simulink model "bh_COMPONENT_3dof_4wheel_car_model"  (R2018a)
settings: Solver=ode45  StartTime=0.0  StopTime=80  FixedStep=0.001  RelTol=1e-5
undefined symbols (not defined in the file): veh, VwW_X_b_L, VwW_X_b_R, VwW_X_f_L, VwW_X_f_R
settings Model: PauseTimes=30  Creator=bhorton  LastModifiedBy=bhorton
settings SolverCC: ZeroCrossControl=EnableAll  ZeroCrossAlgorithm=Adaptive
settings DebuggingCC: SignalInfNanChecking=warning

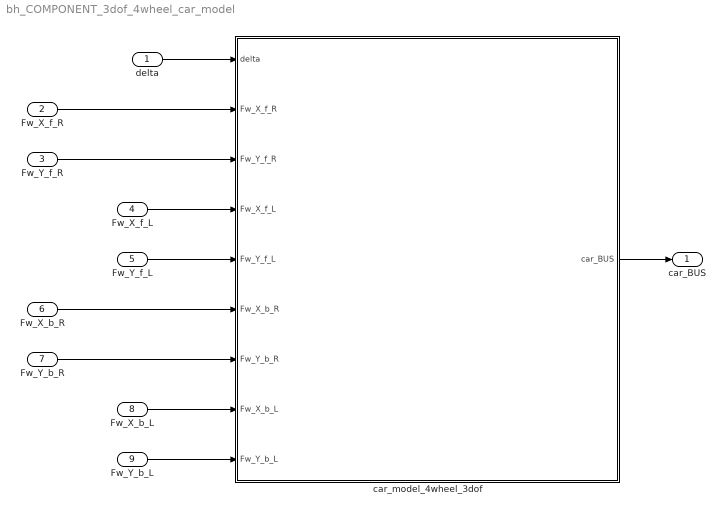
== system bh_COMPONENT_3dof_4wheel_car_model ==
  delta : Inport
  Fw_X_f_R : Inport  Port=2
  Fw_Y_f_R : Inport  Port=3
  Fw_X_f_L : Inport  Port=4
  Fw_Y_f_L : Inport  Port=5
  Fw_X_b_R : Inport  Port=6
  Fw_Y_b_R : Inport  Port=7
  Fw_X_b_L : Inport  Port=8
  Fw_Y_b_L : Inport  Port=9
  car_model_4wheel_3dof : Subsystem  mask{L_f=veh.Lf, L_b=veh.Lb, L_p=veh.Lp, L_d=veh.Ld, m=veh.mass, I_zz=veh.Inertia, v_xB_0=veh.states.init_vel_B_Cx, v_yB_0=veh.states.init_vel_B_Cy, xG_0=veh.states.init_pos_G_Cxy(1), yG_0=veh.states.init_pos_G_Cxy(2), theta_D_0=veh.states.init_theta_vel_rad, theta_0=veh.states.init_theta_pos_rad}
      mask prompts: L_f "Lf  (m)"; L_b "Lb  (m)"; L_p "Lp  (m)"; L_d "Ld  (m)"; m "m  (kg)"; I_zz "I_zz (kg.m^2)"; v_xB_0 "vB_X  (m/sec)"; v_yB_0 "vB_Y (m/sec)"; xG_0 "xG_0 (m)"; yG_0 "yG_0 (m)"; theta_D_0 "theta_dot_0 (rad/sec)"; theta_0 "theta_0  (rad)"
      mask DialogControl DescGroupVar Prompt: 3-dof_4wheel_car_dynamics
      mask DialogControl DescTextVar Prompt: 3-dof 4 wheel car model
      mask DialogControl Container7 Prompt: Diagrams
      mask DialogControl Container12 Prompt: 01
      mask DialogControl Container14 Prompt: 02
      mask DialogControl Container15 Prompt: 03
      mask DialogControl Container24 Prompt: 04
      mask DialogControl Container25 Prompt: 05
      mask DialogControl Container9 Prompt: Geometry
      mask DialogControl Container10 Prompt: Mass
      mask DialogControl Container13 Prompt: States
      mask DialogControl Control5 Prompt: INITIAL velocity in BODY {B}-frame
      mask DialogControl Control6 Prompt: INITIAL position in INERTIAL {G}-frame
      mask DialogControl Control4 Prompt: INITIAL Angular states:
      mask Display: image(imread('bh_CAR_geo_07.JPG'), 'center')
  car_BUS : Outport  OutDataTypeStr=Bus: car_BUS
  wires:
  car_model_4wheel_3dof/1(car_BUS) -> car_BUS/1
  Fw_X_b_L/1 -> car_model_4wheel_3dof/8(Fw_X_b_L)
  Fw_Y_b_L/1 -> car_model_4wheel_3dof/9(Fw_Y_b_L)
  Fw_X_f_R/1 -> car_model_4wheel_3dof/2(Fw_X_f_R)
  Fw_Y_b_R/1 -> car_model_4wheel_3dof/7(Fw_Y_b_R)
  Fw_X_b_R/1 -> car_model_4wheel_3dof/6(Fw_X_b_R)
  Fw_X_f_L/1 -> car_model_4wheel_3dof/4(Fw_X_f_L)
  Fw_Y_f_L/1 -> car_model_4wheel_3dof/5(Fw_Y_f_L)
  delta/1 -> car_model_4wheel_3dof/1(delta)
  Fw_Y_f_R/1 -> car_model_4wheel_3dof/3(Fw_Y_f_R)

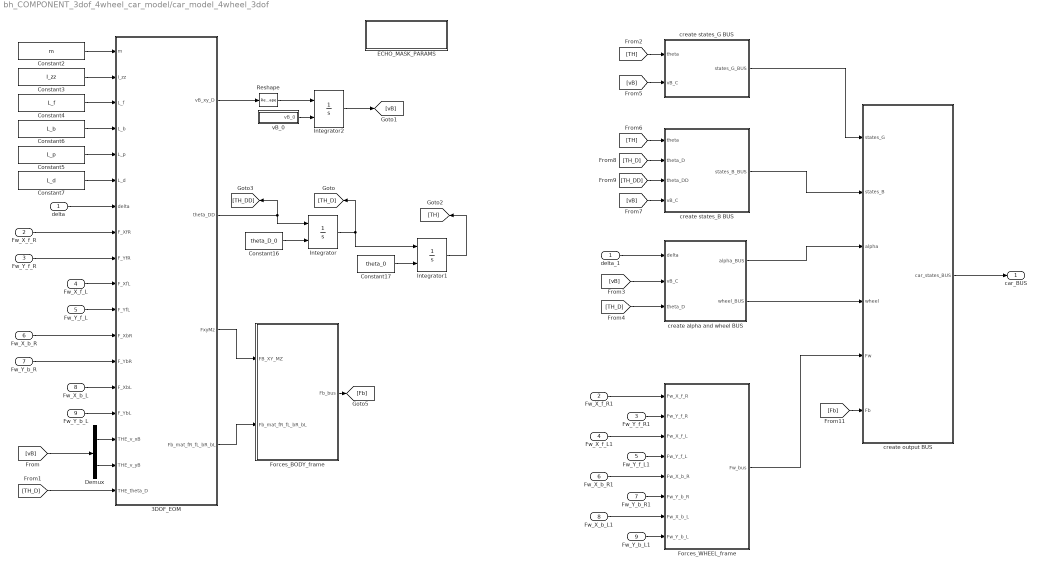
== system bh_COMPONENT_3dof_4wheel_car_model/car_model_4wheel_3dof ==
  delta : Inport
  Fw_X_f_R : Inport  Port=2
  Fw_Y_f_R : Inport  Port=3
  Fw_X_f_L : Inport  Port=4
  Fw_Y_f_L : Inport  Port=5
  Fw_X_b_R : Inport  Port=6
  Fw_Y_b_R : Inport  Port=7
  Fw_X_b_L : Inport  Port=8
  Fw_Y_b_L : Inport  Port=9
  3DOF_EOM : MATLAB Function  TreatAsAtomicUnit=on
  Constant16 : Constant  Value=theta_D_0
  Constant17 : Constant  Value=theta_0
  Constant2 : Constant  Value=m
  Constant3 : Constant  Value=I_zz
  Constant4 : Constant  Value=L_f
  Constant5 : Constant  Value=L_p
  Constant6 : Constant  Value=L_b
  Constant7 : Constant  Value=L_d
  Demux : Demux  Outputs=2
  ECHO_MASK_PARAMS : Subsystem
  Forces_BODY_frame : Subsystem
  Forces_WHEEL_frame : Subsystem
  Fw_X_b_L1 : InportShadow  Port=8
  Fw_X_b_R1 : InportShadow  Port=6
  Fw_X_f_L1 : InportShadow  Port=4
  Fw_X_f_R1 : InportShadow  Port=2
  Fw_Y_b_L1 : InportShadow  Port=9
  Fw_Y_b_R1 : InportShadow  Port=7
  Fw_Y_f_L1 : InportShadow  Port=5
  Fw_Y_f_R1 : InportShadow  Port=3
  Integrator : Integrator  InitialConditionSource=external
  Integrator1 : Integrator  InitialConditionSource=external
  Integrator2 : Integrator  InitialConditionSource=external
  Reshape : Reshape  OutputDimensionality=Column vector (2-D)
  create output BUS : Subsystem
  create alpha and wheel BUS : Subsystem
  create states_B BUS : Subsystem
  create states_G BUS : Subsystem
  delta_1 : InportShadow
  vB_0 : Subsystem
  car_BUS : Outport  OutDataTypeStr=Bus: car_BUS
  wires:
  Fw_X_b_R/1 -> 3DOF_EOM/12(F_XbR)
  3DOF_EOM/1(vB_xy_D) -> Reshape/1
  Integrator/1 -> Integrator1/1, [TH_D]
  Constant3/1 -> 3DOF_EOM/2(I_zz)
  Constant7/1 -> 3DOF_EOM/6(L_d)
  Reshape/1 -> Integrator2/1
  [TH_D] -> create alpha and wheel BUS/3(theta_D)
  delta_1/1 -> create alpha and wheel BUS/1(delta)
  Demux/1 -> 3DOF_EOM/16(THE_v_xB)
  Integrator1/1 -> [TH]
  Fw_X_f_R/1 -> 3DOF_EOM/8(F_XfR)
  [TH] -> create states_B BUS/1(theta)
  create alpha and wheel BUS/1(alpha_BUS) -> create output BUS/3(alpha)
  create states_B BUS/1(states_B_BUS) -> create output BUS/2(states_B)
  Constant4/1 -> 3DOF_EOM/3(L_f)
  Fw_X_f_L/1 -> 3DOF_EOM/10(F_XfL)
  create states_G BUS/1(states_G_BUS) -> create output BUS/1(states_G)
  create output BUS/1(car_states_BUS) -> car_BUS/1
  [TH_D] -> 3DOF_EOM/18(THE_theta_D)
  Constant17/1 -> Integrator1/2
  Constant16/1 -> Integrator/2
  Fw_X_b_L/1 -> 3DOF_EOM/14(F_XbL)
  [vB] -> create states_G BUS/2(vB_C)
  [TH_DD] -> create states_B BUS/3(theta_DD)
  [vB] -> create states_B BUS/4(vB_C)
  [TH] -> create states_G BUS/1(theta)
  [TH_D] -> create states_B BUS/2(theta_D)
  Constant5/1 -> 3DOF_EOM/5(L_p)
  Constant6/1 -> 3DOF_EOM/4(L_b)
  Constant2/1 -> 3DOF_EOM/1(m)
  Fw_Y_b_L/1 -> 3DOF_EOM/15(F_YbL)
  Fw_Y_f_L/1 -> 3DOF_EOM/11(F_YfL)
  Demux/2 -> 3DOF_EOM/17(THE_v_yB)
  Fw_Y_f_R/1 -> 3DOF_EOM/9(F_YfR)
  Integrator2/1 -> [vB]
  vB_0/1(vB_0) -> Integrator2/2
  3DOF_EOM/2(theta_DD) -> [TH_DD], Integrator/1
  [vB] -> Demux/1
  delta/1 -> 3DOF_EOM/7(delta)
  Fw_Y_b_R/1 -> 3DOF_EOM/13(F_YbR)
  [vB] -> create alpha and wheel BUS/2(vB_C)
  create alpha and wheel BUS/2(wheel_BUS) -> create output BUS/4(wheel)
  Fw_Y_f_R1/1 -> Forces_WHEEL_frame/2(Fw_Y_f_R)
  Fw_Y_f_L1/1 -> Forces_WHEEL_frame/4(Fw_Y_f_L)
  Fw_Y_b_R1/1 -> Forces_WHEEL_frame/6(Fw_Y_b_R)
  Fw_Y_b_L1/1 -> Forces_WHEEL_frame/8(Fw_Y_b_L)
  Fw_X_f_L1/1 -> Forces_WHEEL_frame/3(Fw_X_f_L)
  Fw_X_f_R1/1 -> Forces_WHEEL_frame/1(Fw_X_f_R)
  Fw_X_b_R1/1 -> Forces_WHEEL_frame/5(Fw_X_b_R)
  Fw_X_b_L1/1 -> Forces_WHEEL_frame/7(Fw_X_b_L)
  Forces_WHEEL_frame/1(Fw_bus) -> create output BUS/5(Fw)
  3DOF_EOM/3(FxyMz) -> Forces_BODY_frame/1(FB_XY_MZ)
  3DOF_EOM/4(Fb_mat_fR_fL_bR_bL) -> Forces_BODY_frame/2(Fb_mat_fR_fL_bR_bL)
  Forces_BODY_frame/1(Fb_bus) -> [Fb]
  [Fb] -> create output BUS/6(Fb)

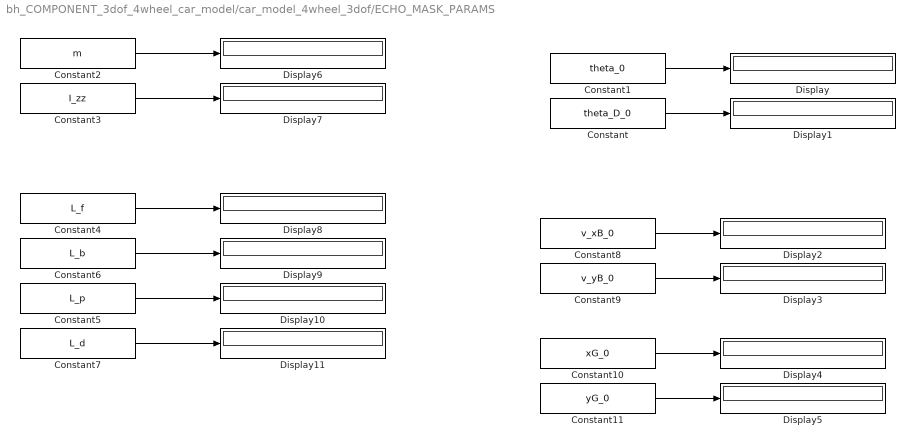
== system bh_COMPONENT_3dof_4wheel_car_model/car_model_4wheel_3dof/ECHO_MASK_PARAMS ==
  Constant : Constant  Value=theta_D_0
  Constant1 : Constant  Value=theta_0
  Constant10 : Constant  Value=xG_0
  Constant11 : Constant  Value=yG_0
  Constant2 : Constant  Value=m
  Constant3 : Constant  Value=I_zz
  Constant4 : Constant  Value=L_f
  Constant5 : Constant  Value=L_p
  Constant6 : Constant  Value=L_b
  Constant7 : Constant  Value=L_d
  Constant8 : Constant  Value=v_xB_0
  Constant9 : Constant  Value=v_yB_0
  Display{,1..11} (12 alike) : Display
  wires:
  Constant1/1 -> Display/1
  Constant/1 -> Display1/1
  Constant8/1 -> Display2/1
  Constant9/1 -> Display3/1
  Constant10/1 -> Display4/1
  Constant11/1 -> Display5/1
  Constant3/1 -> Display7/1
  Constant2/1 -> Display6/1
  Constant4/1 -> Display8/1
  Constant7/1 -> Display11/1
  Constant5/1 -> Display10/1
  Constant6/1 -> Display9/1

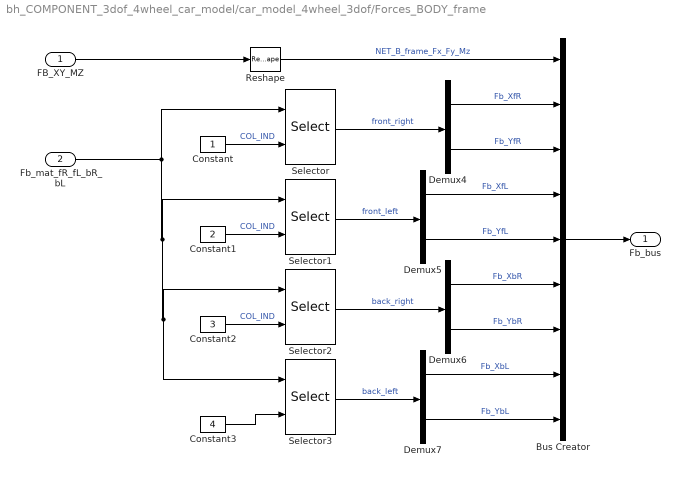
== system bh_COMPONENT_3dof_4wheel_car_model/car_model_4wheel_3dof/Forces_BODY_frame ==
  FB_XY_MZ : Inport
  Fb_mat_fR_fL_bR_bL : Inport  Port=2
  Bus Creator : BusCreator  Inputs=9
  Constant : Constant
  Constant1 : Constant  Value=2
  Constant2 : Constant  Value=3
  Constant3 : Constant  Value=4
  Demux{4..7} (4 alike) : Demux  Outputs=2
  Reshape : Reshape  OutputDimensionality=Column vector (2-D)
  Selector{,1..3} (4 alike) : Selector  NumberOfDimensions=2  InputPortWidth=[2,4]  IndexOptions=Index vector (dialog),Index vector (port)  Indices=[1 2],1  OutputSizes=1,1
  Fb_bus : Outport
  wires:
  Selector/1 -> Demux4/1  "front_right"
  Demux6/2 -> Bus Creator/7  "Fb_YbR"
  Constant1/1 -> Selector1/2  "COL_IND"
  Demux7/1 -> Bus Creator/8  "Fb_XbL"
  Selector1/1 -> Demux5/1  "front_left"
  Selector2/1 -> Demux6/1  "back_right"
  Fb_mat_fR_fL_bR_bL/1 -> Selector/1, Selector3/1, Selector2/1, Selector1/1
  Constant/1 -> Selector/2  "COL_IND"
  Constant2/1 -> Selector2/2  "COL_IND"
  Demux4/1 -> Bus Creator/2  "Fb_XfR"
  Demux6/1 -> Bus Creator/6  "Fb_XbR"
  Demux4/2 -> Bus Creator/3  "Fb_YfR"
  FB_XY_MZ/1 -> Reshape/1
  Demux5/1 -> Bus Creator/4  "Fb_XfL"
  Demux5/2 -> Bus Creator/5  "Fb_YfL"
  Selector3/1 -> Demux7/1  "back_left"
  Demux7/2 -> Bus Creator/9  "Fb_YbL"
  Constant3/1 -> Selector3/2
  Reshape/1 -> Bus Creator/1  "NET_B_frame_Fx_Fy_Mz"
  Bus Creator/1 -> Fb_bus/1

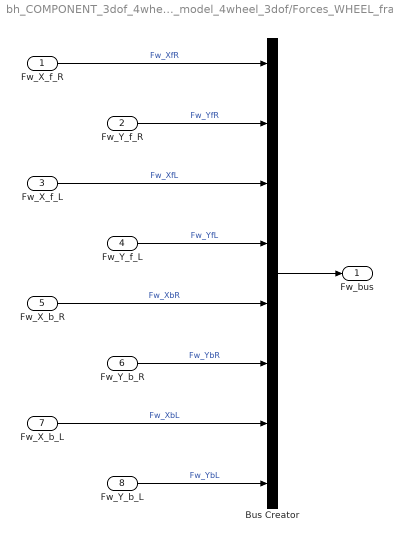
== system bh_COMPONENT_3dof_4wheel_car_model/car_model_4wheel_3dof/Forces_WHEEL_frame ==
  Fw_X_f_R : Inport
  Fw_Y_f_R : Inport  Port=2
  Fw_X_f_L : Inport  Port=3
  Fw_Y_f_L : Inport  Port=4
  Fw_X_b_R : Inport  Port=5
  Fw_Y_b_R : Inport  Port=6
  Fw_X_b_L : Inport  Port=7
  Fw_Y_b_L : Inport  Port=8
  Bus Creator : BusCreator  Inputs=8
  Fw_bus : Outport
  wires:
  Fw_Y_f_R/1 -> Bus Creator/2  "Fw_YfR"
  Fw_X_f_R/1 -> Bus Creator/1  "Fw_XfR"
  Fw_Y_b_R/1 -> Bus Creator/6  "Fw_YbR"
  Fw_X_b_R/1 -> Bus Creator/5  "Fw_XbR"
  Fw_X_f_L/1 -> Bus Creator/3  "Fw_XfL"
  Fw_Y_f_L/1 -> Bus Creator/4  "Fw_YfL"
  Fw_X_b_L/1 -> Bus Creator/7  "Fw_XbL"
  Fw_Y_b_L/1 -> Bus Creator/8  "Fw_YbL"
  Bus Creator/1 -> Fw_bus/1

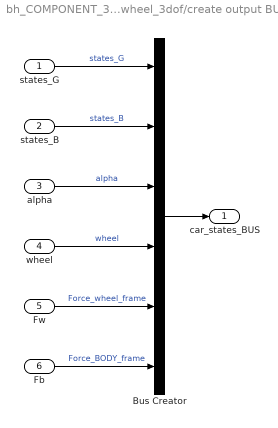
== system bh_COMPONENT_3dof_4wheel_car_model/car_model_4wheel_3dof/create output BUS ==
  states_G : Inport
  states_B : Inport  Port=2
  alpha : Inport  Port=3
  wheel : Inport  Port=4
  Fw : Inport  Port=5
  Fb : Inport  Port=6
  Bus Creator : BusCreator  Inputs=6
  car_states_BUS : Outport
  wires:
  alpha/1 -> Bus Creator/3  "alpha"
  states_B/1 -> Bus Creator/2  "states_B"
  states_G/1 -> Bus Creator/1  "states_G"
  Bus Creator/1 -> car_states_BUS/1
  wheel/1 -> Bus Creator/4  "wheel"
  Fw/1 -> Bus Creator/5  "Force_wheel_frame"
  Fb/1 -> Bus Creator/6  "Force_BODY_frame"

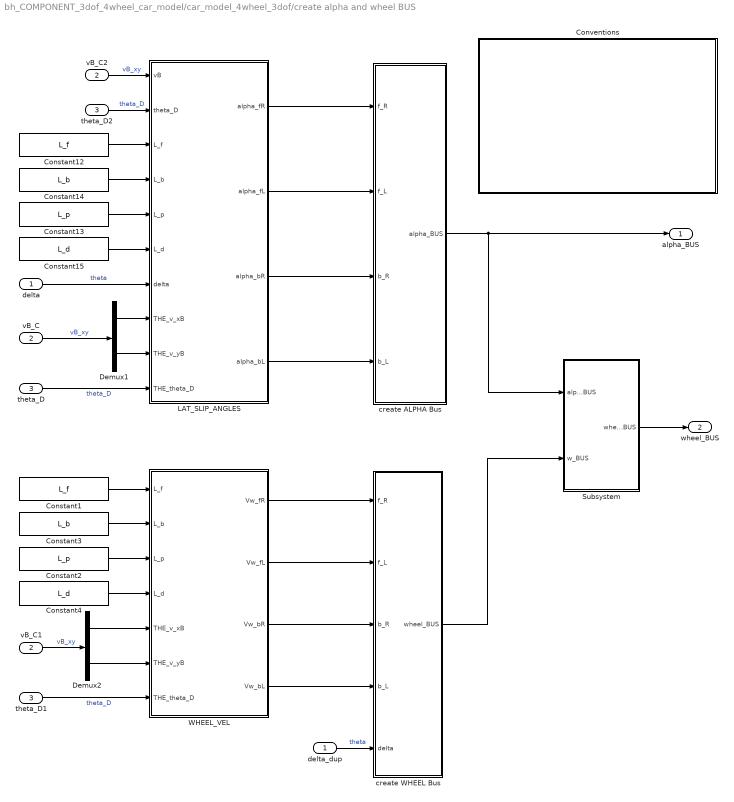
== system bh_COMPONENT_3dof_4wheel_car_model/car_model_4wheel_3dof/create alpha and wheel BUS ==
  delta : Inport
  vB_C : Inport  Port=2
  theta_D : Inport  Port=3
  Constant1 : Constant  Value=L_f
  Constant12 : Constant  Value=L_f
  Constant13 : Constant  Value=L_p
  Constant14 : Constant  Value=L_b
  Constant15 : Constant  Value=L_d
  Constant2 : Constant  Value=L_p
  Constant3 : Constant  Value=L_b
  Constant4 : Constant  Value=L_d
  Conventions : Subsystem
  Demux1 : Demux  Outputs=2
  Demux2 : Demux  Outputs=2
  LAT_SLIP_ANGLES : MATLAB Function  TreatAsAtomicUnit=on
  Subsystem : Subsystem
  WHEEL_VEL : MATLAB Function  TreatAsAtomicUnit=on
  create ALPHA Bus : Subsystem
  create WHEEL Bus : Subsystem
  delta_dup : InportShadow
  theta_D1 : InportShadow  Port=3
  theta_D2 : InportShadow  Port=3
  vB_C1 : InportShadow  Port=2
  vB_C2 : InportShadow  Port=2
  alpha_BUS : Outport
  wheel_BUS : Outport  Port=2
  wires:
  Constant15/1 -> LAT_SLIP_ANGLES/6(L_d)
  Constant13/1 -> LAT_SLIP_ANGLES/5(L_p)
  Constant14/1 -> LAT_SLIP_ANGLES/4(L_b)
  Constant12/1 -> LAT_SLIP_ANGLES/3(L_f)
  Demux1/2 -> LAT_SLIP_ANGLES/9(THE_v_yB)
  Demux1/1 -> LAT_SLIP_ANGLES/8(THE_v_xB)
  vB_C/1 -> Demux1/1  "vB_xy"
  delta/1 -> LAT_SLIP_ANGLES/7(delta)  "theta"
  Constant1/1 -> WHEEL_VEL/1(L_f)
  Constant3/1 -> WHEEL_VEL/2(L_b)
  Constant2/1 -> WHEEL_VEL/3(L_p)
  Constant4/1 -> WHEEL_VEL/4(L_d)
  Demux2/2 -> WHEEL_VEL/6(THE_v_yB)
  Demux2/1 -> WHEEL_VEL/5(THE_v_xB)
  vB_C1/1 -> Demux2/1  "vB_xy"
  theta_D1/1 -> WHEEL_VEL/7(THE_theta_D)  "theta_D"
  WHEEL_VEL/1(Vw_fR) -> create WHEEL Bus/1(f_R)
  WHEEL_VEL/2(Vw_fL) -> create WHEEL Bus/2(f_L)
  WHEEL_VEL/3(Vw_bR) -> create WHEEL Bus/3(b_R)
  WHEEL_VEL/4(Vw_bL) -> create WHEEL Bus/4(b_L)
  create ALPHA Bus/1(alpha_BUS) -> alpha_BUS/1, Subsystem/1(alpha_BUS)
  create WHEEL Bus/1(wheel_BUS) -> Subsystem/2(w_BUS)
  Subsystem/1(wheel_BUS) -> wheel_BUS/1
  delta_dup/1 -> create WHEEL Bus/5(delta)  "theta"
  LAT_SLIP_ANGLES/3(alpha_bR) -> create ALPHA Bus/3(b_R)
  LAT_SLIP_ANGLES/2(alpha_fL) -> create ALPHA Bus/2(f_L)
  LAT_SLIP_ANGLES/4(alpha_bL) -> create ALPHA Bus/4(b_L)
  LAT_SLIP_ANGLES/1(alpha_fR) -> create ALPHA Bus/1(f_R)
  theta_D2/1 -> LAT_SLIP_ANGLES/2(theta_D)  "theta_D"
  vB_C2/1 -> LAT_SLIP_ANGLES/1(vB)  "vB_xy"
  theta_D/1 -> LAT_SLIP_ANGLES/10(THE_theta_D)  "theta_D"

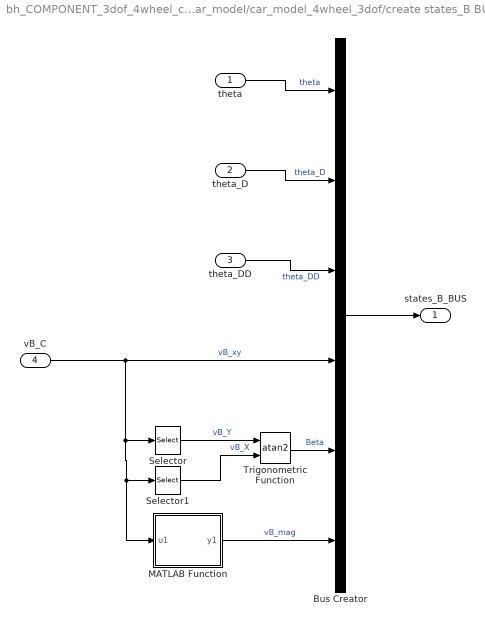
== system bh_COMPONENT_3dof_4wheel_car_model/car_model_4wheel_3dof/create states_B BUS ==
  theta : Inport
  theta_D : Inport  Port=2
  theta_DD : Inport  Port=3
  vB_C : Inport  Port=4
  Bus Creator : BusCreator  Inputs=6
  MATLAB Function : MATLAB Function  TreatAsAtomicUnit=on
  Selector : Selector  InputPortWidth=2  IndexOptions=Index vector (dialog)  Indices=2  OutputSizes=1
  Selector1 : Selector  InputPortWidth=2  IndexOptions=Index vector (dialog)  Indices=1  OutputSizes=1
  Trigonometric Function : Trigonometry  Operator=atan2
  states_B_BUS : Outport
  wires:
  Bus Creator/1 -> states_B_BUS/1
  vB_C/1 -> Selector/1, MATLAB Function/1(u1), Selector1/1, Bus Creator/4  "vB_xy"
  theta/1 -> Bus Creator/1  "theta"
  theta_D/1 -> Bus Creator/2  "theta_D"
  theta_DD/1 -> Bus Creator/3  "theta_DD"
  Trigonometric Function/1 -> Bus Creator/5  "Beta"
  Selector/1 -> Trigonometric Function/1  "vB_Y"
  MATLAB Function/1(y1) -> Bus Creator/6  "vB_mag"
  Selector1/1 -> Trigonometric Function/2  "vB_X"

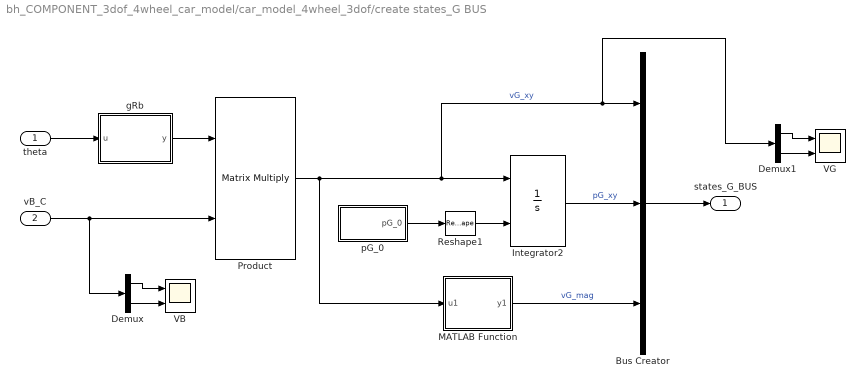
== system bh_COMPONENT_3dof_4wheel_car_model/car_model_4wheel_3dof/create states_G BUS ==
  theta : Inport
  vB_C : Inport  Port=2
  Bus Creator : BusCreator  Inputs=3
  Demux : Demux  Outputs=2
  Demux1 : Demux  Outputs=2
  Integrator2 : Integrator  InitialConditionSource=external
  MATLAB Function : MATLAB Function  TreatAsAtomicUnit=on
  Product : Product  Multiplication=Matrix(*)
  Reshape1 : Reshape  OutputDimensionality=Column vector (2-D)
  VB : Scope  NumInputPorts=2
  VG : Scope  NumInputPorts=2
  gRb : MATLAB Function  TreatAsAtomicUnit=on
  pG_0 : Subsystem
  states_G_BUS : Outport
  wires:
  theta/1 -> gRb/1(u)
  Integrator2/1 -> Bus Creator/2  "pG_xy"
  Reshape1/1 -> Integrator2/2
  Bus Creator/1 -> states_G_BUS/1
  pG_0/1(pG_0) -> Reshape1/1
  gRb/1(y) -> Product/1
  vB_C/1 -> Demux/1, Product/2
  Product/1 -> MATLAB Function/1(u1), Demux1/1, Bus Creator/1, Integrator2/1  "vG_xy"
  MATLAB Function/1(y1) -> Bus Creator/3  "vG_mag"
  Demux/1 -> VB/1
  Demux/2 -> VB/2
  Demux1/2 -> VG/2
  Demux1/1 -> VG/1

== system bh_COMPONENT_3dof_4wheel_car_model/car_model_4wheel_3dof/vB_0 ==
  Constant8 : Constant  Value=v_xB_0
  Constant9 : Constant  Value=v_yB_0
  Mux : Mux  Inputs=2
  Reshape : Reshape  OutputDimensionality=Column vector (2-D)
  vB_0 : Outport
  wires:
  Constant9/1 -> Mux/2
  Reshape/1 -> vB_0/1
  Mux/1 -> Reshape/1
  Constant8/1 -> Mux/1

== system bh_COMPONENT_3dof_4wheel_car_model/car_model_4wheel_3dof/create alpha and wheel BUS/Conventions ==

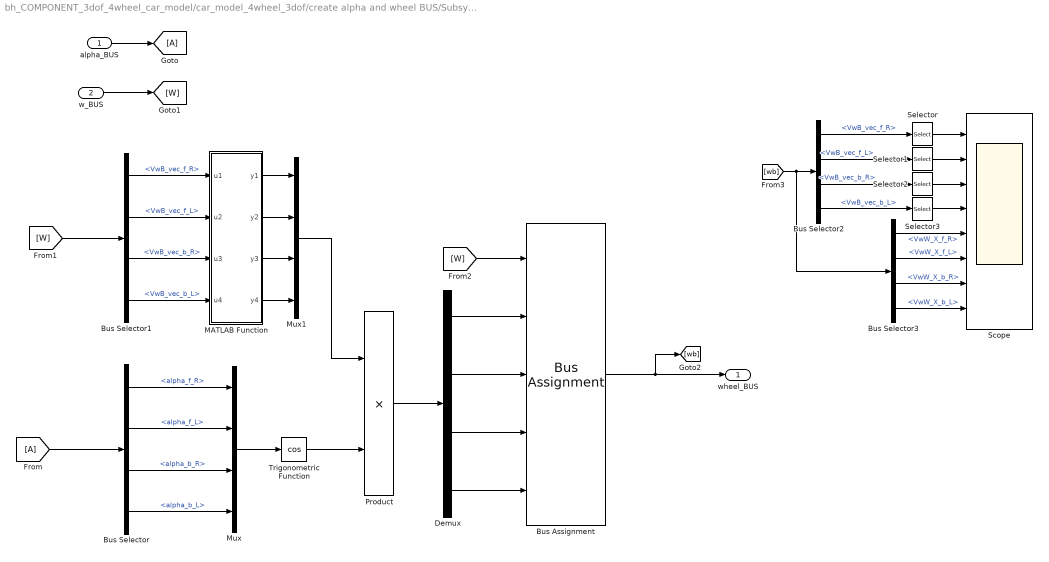
== system bh_COMPONENT_3dof_4wheel_car_model/car_model_4wheel_3dof/create alpha and wheel BUS/Subsystem ==
  alpha_BUS : Inport
  w_BUS : Inport  Port=2
  Bus Assignment : BusAssignment  AssignedSignals=VwW_X_f_R,VwW_X_f_L,VwW_X_b_R,VwW_X_b_L
  Bus Selector : BusSelector  OutputSignals=alpha_f_R,alpha_f_L,alpha_b_R,alpha_b_L
  Bus Selector1 : BusSelector  OutputSignals=VwB_vec_f_R,VwB_vec_f_L,VwB_vec_b_R,VwB_vec_b_L
  Bus Selector2 : BusSelector  OutputSignals=VwB_vec_f_R,VwB_vec_f_L,VwB_vec_b_R,VwB_vec_b_L
  Bus Selector3 : BusSelector  OutputSignals=VwW_X_f_R,VwW_X_f_L,VwW_X_b_R,VwW_X_b_L
  Demux : Demux
  MATLAB Function : MATLAB Function  TreatAsAtomicUnit=on
  Mux : Mux
  Mux1 : Mux
  Product : Product
  Scope : Scope  NumInputPorts=8
  Selector{,1..3} (4 alike) : Selector  InputPortWidth=2  IndexOptions=Index vector (dialog)  Indices=1  OutputSizes=1
  Trigonometric Function : Trigonometry  Operator=cos
  wheel_BUS : Outport
  wires:
  Bus Assignment/1 -> [wb], wheel_BUS/1
  alpha_BUS/1 -> [A]
  [A] -> Bus Selector/1
  Bus Selector/1 -> Mux/1  "<alpha_f_R>"
  Bus Selector/2 -> Mux/2  "<alpha_f_L>"
  Bus Selector/3 -> Mux/3  "<alpha_b_R>"
  Bus Selector/4 -> Mux/4  "<alpha_b_L>"
  Mux/1 -> Trigonometric Function/1
  w_BUS/1 -> [W]
  [W] -> Bus Selector1/1
  Bus Selector1/1 -> MATLAB Function/1(u1)  "<VwB_vec_f_R>"
  Bus Selector1/2 -> MATLAB Function/2(u2)  "<VwB_vec_f_L>"
  Bus Selector1/3 -> MATLAB Function/3(u3)  "<VwB_vec_b_R>"
  Bus Selector1/4 -> MATLAB Function/4(u4)  "<VwB_vec_b_L>"
  MATLAB Function/1(y1) -> Mux1/1
  MATLAB Function/2(y2) -> Mux1/2
  MATLAB Function/3(y3) -> Mux1/3
  MATLAB Function/4(y4) -> Mux1/4
  Demux/1 -> Bus Assignment/2
  Demux/2 -> Bus Assignment/3
  Demux/3 -> Bus Assignment/4
  Demux/4 -> Bus Assignment/5
  Product/1 -> Demux/1
  Trigonometric Function/1 -> Product/2
  Mux1/1 -> Product/1
  [W] -> Bus Assignment/1
  Bus Selector2/1 -> Selector/1  "<VwB_vec_f_R>"
  Bus Selector2/2 -> Selector1/1  "<VwB_vec_f_L>"
  Bus Selector2/3 -> Selector2/1  "<VwB_vec_b_R>"
  Bus Selector2/4 -> Selector3/1  "<VwB_vec_b_L>"
  [wb] -> Bus Selector3/1, Bus Selector2/1
  Selector/1 -> Scope/1
  Selector3/1 -> Scope/4
  Selector2/1 -> Scope/3
  Selector1/1 -> Scope/2
  Bus Selector3/1 -> Scope/5  "<VwW_X_f_R>"
  Bus Selector3/2 -> Scope/6  "<VwW_X_f_L>"
  Bus Selector3/3 -> Scope/7  "<VwW_X_b_R>"
  Bus Selector3/4 -> Scope/8  "<VwW_X_b_L>"

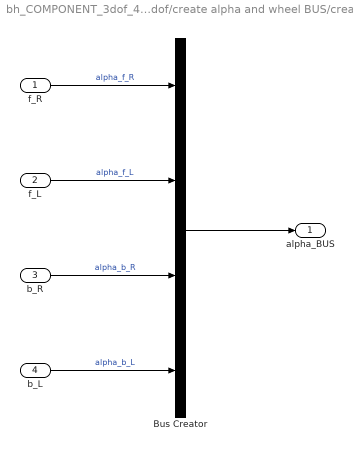
== system bh_COMPONENT_3dof_4wheel_car_model/car_model_4wheel_3dof/create alpha and wheel BUS/create ALPHA Bus ==
  f_R : Inport
  f_L : Inport  Port=2
  b_R : Inport  Port=3
  b_L : Inport  Port=4
  Bus Creator : BusCreator  Inputs=4
  alpha_BUS : Outport
  wires:
  f_R/1 -> Bus Creator/1  "alpha_f_R"
  f_L/1 -> Bus Creator/2  "alpha_f_L"
  b_R/1 -> Bus Creator/3  "alpha_b_R"
  b_L/1 -> Bus Creator/4  "alpha_b_L"
  Bus Creator/1 -> alpha_BUS/1

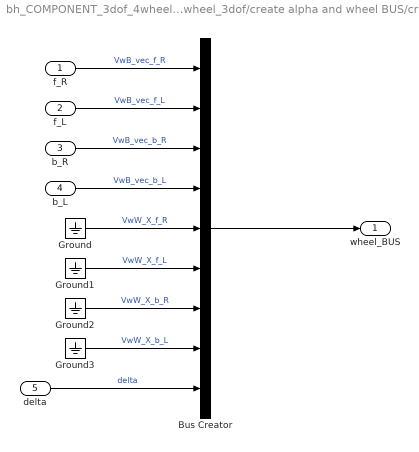
== system bh_COMPONENT_3dof_4wheel_car_model/car_model_4wheel_3dof/create alpha and wheel BUS/create WHEEL Bus ==
  f_R : Inport
  f_L : Inport  Port=2
  b_R : Inport  Port=3
  b_L : Inport  Port=4
  delta : Inport  Port=5
  Bus Creator : BusCreator  Inputs=9
  Ground{,1..3} (4 alike) : Ground
  wheel_BUS : Outport
  wires:
  f_R/1 -> Bus Creator/1  "VwB_vec_f_R"
  f_L/1 -> Bus Creator/2  "VwB_vec_f_L"
  b_R/1 -> Bus Creator/3  "VwB_vec_b_R"
  b_L/1 -> Bus Creator/4  "VwB_vec_b_L"
  Bus Creator/1 -> wheel_BUS/1
  Ground/1 -> Bus Creator/5  "VwW_X_f_R"
  Ground1/1 -> Bus Creator/6  "VwW_X_f_L"
  Ground2/1 -> Bus Creator/7  "VwW_X_b_R"
  Ground3/1 -> Bus Creator/8  "VwW_X_b_L"
  delta/1 -> Bus Creator/9  "delta"

== system bh_COMPONENT_3dof_4wheel_car_model/car_model_4wheel_3dof/create states_G BUS/pG_0 ==
  Constant10 : Constant  Value=xG_0
  Constant11 : Constant  Value=yG_0
  Mux : Mux  Inputs=2
  Reshape : Reshape  OutputDimensionality=Column vector (2-D)
  pG_0 : Outport
  wires:
  Constant11/1 -> Mux/2
  Reshape/1 -> pG_0/1
  Mux/1 -> Reshape/1
  Constant10/1 -> Mux/1

== matlab function bh_COMPONENT_3dof_4wheel_car_model/car_model_4wheel_3dof/create states_G BUS/MATLAB Function ==
  data: u1 input; y1 output
function y1  = mag(u1) %#codegen

y1 = norm(u1);

end

== matlab function bh_COMPONENT_3dof_4wheel_car_model/car_model_4wheel_3dof/create states_B BUS/MATLAB Function ==
  data: u1 input; y1 output
function y1  = mag(u1) %#codegen

y1 = norm(u1);

end

== matlab function bh_COMPONENT_3dof_4wheel_car_model/car_model_4wheel_3dof/create states_G BUS/gRb ==
  data: u input; y output
function y = fcn(u)

y = [ cos(u), -sin(u);
      sin(u),  cos(u) ];
  
end

== matlab function bh_COMPONENT_3dof_4wheel_car_model/car_model_4wheel_3dof/create alpha and wheel BUS/LAT_SLIP_ANGLES ==
  data: vB input; theta_D input; L_f input; alpha_fR output; L_b input; L_p input; L_d input; delta input; THE_v_xB input; THE_v_yB input; THE_theta_D input; alpha_fL output; alpha_bR output; alpha_bL output
function [alpha_fR,alpha_fL,alpha_bR,alpha_bL] = LAT_SLIP_ANGLES(vB, theta_D, L_f,L_b,L_p,L_d,delta,THE_v_xB,THE_v_yB,THE_theta_D)
%#codegen

%#codegen

% guard against the 0/0 instance associated with the car being stationary,
% ie:
%     vB_x = vB_y = theta_dot = 0

alpha_fR = 0;
alpha_fL = 0;
alpha_bR = 0;
alpha_bL = 0;

V_MAG       = norm(vB);
vB_X        = vB(1);
APPROX_ZERO = 1e-5;

% SPECIAL CASE #1:
% if BOTH trans and rotational velocities are BOTH zero
% then we're probably stationary

if(V_MAG < APPROX_ZERO  &  abs(theta_D) < APPROX_ZERO)
    alpha_fR = 0;
    alpha_fL = 0;
    alpha_bR = 0;
    alpha_bL = 0;
    return  % RETURN
end

% define the X and Y velocities of each wheel(in the car body frame)
% our vector will be ordered according to:  
%    1.) front_RIGHT
%    2.) front_LEFT
%    3.) back_RIGHT
%    4.) back_LEFT

vY = zeros(4,1);  vX = zeros(4,1);  

vY(1) = (THE_v_yB+L_f.*THE_theta_D);   vX(1) = (THE_v_xB+L_d.*THE_theta_D);
vY(2) = (THE_v_yB+L_f.*THE_theta_D);   vX(2) = (THE_v_xB-L_p.*THE_theta_D);
vY(3) = (THE_v_yB-L_b.*THE_theta_D);   vX(3) = (THE_v_xB+L_d.*THE_theta_D);
vY(4) = (THE_v_yB-L_b.*THE_theta_D);   vX(4) = (THE_v_xB-L_p.*THE_theta_D);

% The car is moving 
if(vB_X > 0)  % moving FORWARD
   alpha_fR = delta -atan(vY(1) / vX(1));  % 1
   alpha_fL = delta -atan(vY(2) / vX(2));  % 2
   alpha_bR =       -atan(vY(3) / vX(3));  % 3
   alpha_bL =       -atan(vY(4) / vX(4));  % 4
else % moving BACKWARDS
   phi_rad            = atan2(vY, vX);  % [-pi, pi]
   phi_rad_star_2PI   = LOC_convert_to_2pi_range( phi_rad );
   delta_rad_star_2PI = LOC_convert_to_2pi_range( (delta + pi) );
   
   % process the FRONT wheels    
   alpha_fR = -1*(delta_rad_star_2PI - phi_rad_star_2PI(1));
   alpha_fL = -1*(delta_rad_star_2PI - phi_rad_star_2PI(2));
   
   % process the BACK wheels 
   alpha_bR = -1*(pi - phi_rad_star_2PI(3));
   alpha_bL = -1*(pi - phi_rad_star_2PI(4));
end  
   
end % LAT_SLIP_ANGLES()
%_#########################################################################
function my_out = LOC_convert_to_2pi_range( some_rad_vec )

   N = length(some_rad_vec);
   my_out = zeros(size(some_rad_vec));
   
   for kk=1:N
       if(some_rad_vec(kk)<0)
         my_out(kk) = 2*pi +   some_rad_vec(kk);
       else
         my_out(kk) = some_rad_vec(kk);  
       end
   end
end % LOC_convert_to_2pi_range()

== matlab function bh_COMPONENT_3dof_4wheel_car_model/car_model_4wheel_3dof/create alpha and wheel BUS/WHEEL_VEL ==
  data: L_f input; Vw_fR output; L_b input; L_p input; L_d input; THE_v_xB input; THE_v_yB input; THE_theta_D input; Vw_fL output; Vw_bR output; Vw_bL output
function [Vw_fR,Vw_fL,Vw_bR,Vw_bL] = WHEEL_VEL(L_f,L_b,L_p,L_d,THE_v_xB,THE_v_yB,THE_theta_D)
%#codegen

%    This function was generated by the Symbolic Math Toolbox version 8.0.
%    22-Nov-2017 09:16:58

Vw_fR = [THE_v_xB+L_d.*THE_theta_D;THE_v_yB+L_f.*THE_theta_D];
if nargout > 1
    Vw_fL = [THE_v_xB-L_p.*THE_theta_D;THE_v_yB+L_f.*THE_theta_D];
end
if nargout > 2
    Vw_bR = [THE_v_xB+L_d.*THE_theta_D;THE_v_yB-L_b.*THE_theta_D];
end
if nargout > 3
    Vw_bL = [THE_v_xB-L_p.*THE_theta_D;THE_v_yB-L_b.*THE_theta_D];
end

== matlab function bh_COMPONENT_3dof_4wheel_car_model/car_model_4wheel_3dof/create alpha and wheel BUS/Subsystem/MATLAB Function ==
  data: u1 input; y1 output; u2 input; u3 input; u4 input; y2 output; y3 output; y4 output
function [y1,y2,y3,y4] = mag(u1,u2,u3,u4) %#codegen

y1 = norm(u1);
y2 = norm(u2);
y3 = norm(u3);
y4 = norm(u4);

end

== matlab function bh_COMPONENT_3dof_4wheel_car_model/car_model_4wheel_3dof/3DOF_EOM ==
  data: m input; vB_xy_D output; I_zz input; L_f input; L_b input; L_p input; L_d input; delta input; F_XfR input; F_YfR input; F_XfL input; F_YfL input; F_XbR input; F_YbR input; F_XbL input; F_YbL input; THE_v_xB input; THE_v_yB input; THE_theta_D input; theta_DD output; FxyMz output; Fb_mat_fR_fL_bR_bL output
function [vB_xy_D,theta_DD,FxyMz,Fb_mat_fR_fL_bR_bL] =  DOF_EOM(m,I_zz,L_f,L_b,L_p,L_d,delta,F_XfR,F_YfR,F_XfL,F_YfL,F_XbR,F_YbR,F_XbL,F_YbL,THE_v_xB,THE_v_yB,THE_theta_D)
%#codegen

%    This function was generated by the Symbolic Math Toolbox version 8.0.
%    23-Nov-2017 12:29:31

vB_xy_D = [(F_XbL+F_XbR+F_XfL.*cos(delta)+F_XfR.*cos(delta)-F_YfL.*sin(delta)-F_YfR.*sin(delta)+THE_v_yB.*THE_theta_D.*m)./m;(F_YbL+F_YbR+F_YfL.*cos(delta)+F_YfR.*cos(delta)+F_XfL.*sin(delta)+F_XfR.*sin(delta)-THE_v_xB.*THE_theta_D.*m)./m];
if nargout > 1
    theta_DD = (-F_YbL.*L_b-F_YbR.*L_b+F_XbR.*L_d-F_XbL.*L_p+F_XfR.*L_d.*cos(delta)+F_YfL.*L_f.*cos(delta)+F_YfR.*L_f.*cos(delta)-F_XfL.*L_p.*cos(delta)-F_YfR.*L_d.*sin(delta)+F_XfL.*L_f.*sin(delta)+F_XfR.*L_f.*sin(delta)+F_YfL.*L_p.*sin(delta))./I_zz;
end
if nargout > 2
    FxyMz = [F_XbL+F_XbR+F_XfL.*cos(delta)+F_XfR.*cos(delta)-F_YfL.*sin(delta)-F_YfR.*sin(delta);F_YbL+F_YbR+F_YfL.*cos(delta)+F_YfR.*cos(delta)+F_XfL.*sin(delta)+F_XfR.*sin(delta);-F_YbL.*L_b-F_YbR.*L_b+F_XbR.*L_d-F_XbL.*L_p+L_d.*(F_XfR.*cos(delta)-F_YfR.*sin(delta))+L_f.*(F_YfL.*cos(delta)+F_XfL.*sin(delta))+L_f.*(F_YfR.*cos(delta)+F_XfR.*sin(delta))-L_p.*(F_XfL.*cos(delta)-F_YfL.*sin(delta))];
end
if nargout > 3
    Fb_mat_fR_fL_bR_bL = reshape([F_XfR.*cos(delta)-F_YfR.*sin(delta),F_YfR.*cos(delta)+F_XfR.*sin(delta),F_XfL.*cos(delta)-F_YfL.*sin(delta),F_YfL.*cos(delta)+F_XfL.*sin(delta),F_XbR,F_YbR,F_XbL,F_YbL],[2,4]);
end
